simulink model "Flight_Controllers"  (R2024a)
settings: Solver=VariableStepAuto  StartTime=0.0  StopTime=tFinal  FixedStep=0.02  RelTol=1e-3
values from neighbouring files (symbols this model uses):
  bOmega = -bThrust/mThrust    (= 168.963839792)    [Load_VehicleParams.m]
  Cant_cosine_Loss = cos(fanCantAngle)    [Load_VehicleParams.m]
  g = 9.807    [Load_VehicleParams.m]
  g_Offset = 5/6    (= 0.833333333333)    [Load_VehicleParams.m]
  Kd_LatPos = -0.04577    [Load_Controller_Gains_1.m]    (also in Load_Controller_Gains_13.m = -0.1; Load_Controller_Gains_2.m = 0.642; Load_Controller_Gains_3.m = -0.103; Load_Controller_Gains_4.m = 0)
  Kd_LatVel = 0    [Load_Controller_Gains_4.m]
  Kd_Pitch = 14.4    [Load_Controller_Gains_1.m]    (also in Load_Controller_Gains_13.m = 40; Load_Controller_Gains_2.m = 33; Load_Controller_Gains_3.m = 40; Load_Controller_Gains_4.m = 78.1)
  Ki_LatPos = -9.22e-6    (= -9.22e-06)    [Load_Controller_Gains_1.m]    (also in Load_Controller_Gains_13.m = 0.001; Load_Controller_Gains_2.m = 0.0199; Load_Controller_Gains_3.m = 0; Load_Controller_Gains_4.m = 0)
  Ki_LatVel = -0.00284    [Load_Controller_Gains_1.m]    (also in Load_Controller_Gains_2.m = -0.0122; Load_Controller_Gains_4.m = 0)
  Ki_Pitch = 3.17    [Load_Controller_Gains_4.m]
  Kp_LatPos = -0.0024    [Load_Controller_Gains_1.m]    (also in Load_Controller_Gains_13.m = -0.0248; Load_Controller_Gains_2.m = 1.53; Load_Controller_Gains_3.m = -0.0175; Load_Controller_Gains_4.m = 0.413)
  Kp_LatVel = -0.0296    [Load_Controller_Gains_1.m]    (also in Load_Controller_Gains_2.m = -0.059; Load_Controller_Gains_4.m = -0.291)
  Kp_Pitch = 5.36    [Load_Controller_Gains_1.m]    (also in Load_Controller_Gains_13.m = 38; Load_Controller_Gains_2.m = 24.8; Load_Controller_Gains_3.m = 38; Load_Controller_Gains_4.m = 43.7)
  mOmega = 1/mThrust    (= 1.62153397114)    [Load_VehicleParams.m]
  N_LatPos = 54.3    [Load_Controller_Gains_1.m]    (also in Load_Controller_Gains_13.m = 120; Load_Controller_Gains_2.m = 15.8; Load_Controller_Gains_3.m = 12; Load_Controller_Gains_4.m = 0)
  N_LatVel = 0    [Load_Controller_Gains_4.m]
  N_Pitch = 18.2    [Load_Controller_Gains_1.m]    (also in Load_Controller_Gains_13.m = 550; Load_Controller_Gains_2.m = 109; Load_Controller_Gains_3.m = 550; Load_Controller_Gains_4.m = 1115)
  nFans = 4    [Load_VehicleParams.m]
  pitch_Cmd_Limit = 7*pi/180    (= 0.12217304764)    [Load_Controller_Gains_13.m]    (also in Load_Controller_Gains_2.m = 0.10471975512; Load_Controller_Gains_3.m; Load_Controller_Gains_4.m)
  tau_LatPos = 0.2    [Load_Controller_Gains_1.m]    (also in Load_Controller_Gains_2.m = 0.01)
  tau_vCmd = 0.01    [Load_Controller_Gains_2.m]    (also in Load_Controller_Gains_4.m = 0.1)
  tau_xCmd = 0.2    [Load_Controller_Gains_3.m]
  Ts_Control = 1/50    (= 0.02)    [run_Lander_GNC_MonteCarloSim.m]
  vCmd_Integr_Limit = 0.25    [Load_Controller_Gains_2.m]
  velCmd_Limit = 2    [Load_Controller_Gains_2.m]    (also in Load_Controller_Gains_4.m = 0.12217304764)
undefined symbols (not defined in the file or in its folder): den_Gc_z_Pitch, den_Gc_z_Pos, num_Gc_z_Pitch, num_Gc_z_Pos, posCntrl_Integr_Limit
libraries: slpidlib x17
(part 1 of 3)
settings Model: Creator=mhannan  LastModifiedBy=mhann
settings SolverCC: AlgebraicLoopSolver=TrustRegion
settings DataIOCC: SaveOutput=off  SaveTime=off
settings OptimizationCC: DefaultParameterBehavior=Inlined  EnhancedBackFolding=on  PassReuseOutputArgsThreshold=0  OptimizeBlockOrder=speed  DifferentSizesBufferReuse=on
settings DebuggingCC: ParameterTunabilityLossMsg=error  UnconnectedInputMsg=warning  UnconnectedOutputMsg=warning  UnconnectedLineMsg=warning  ArithmeticOperatorsInVariantConditions=warning
settings ModelReferenceCC: EnableRefExpFcnMdlSchedulingChecks=on
settings SFSimCC: SimUseLocalCustomCode=off  MATLABDynamicMemAlloc=off  CustomCodeUndefinedFunction=UseInterfaceOnly
settings RTWCC: RTWUseLocalCustomCode=off  GPUComputeCapability=3.5
settings CodeAppCC: ForceParamTrailComments=on  OperatorAnnotations=on

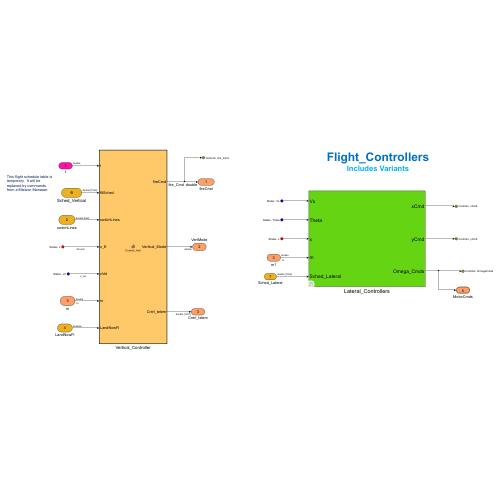
[thumbnail: Simulink's stored preview of the top-level diagram]
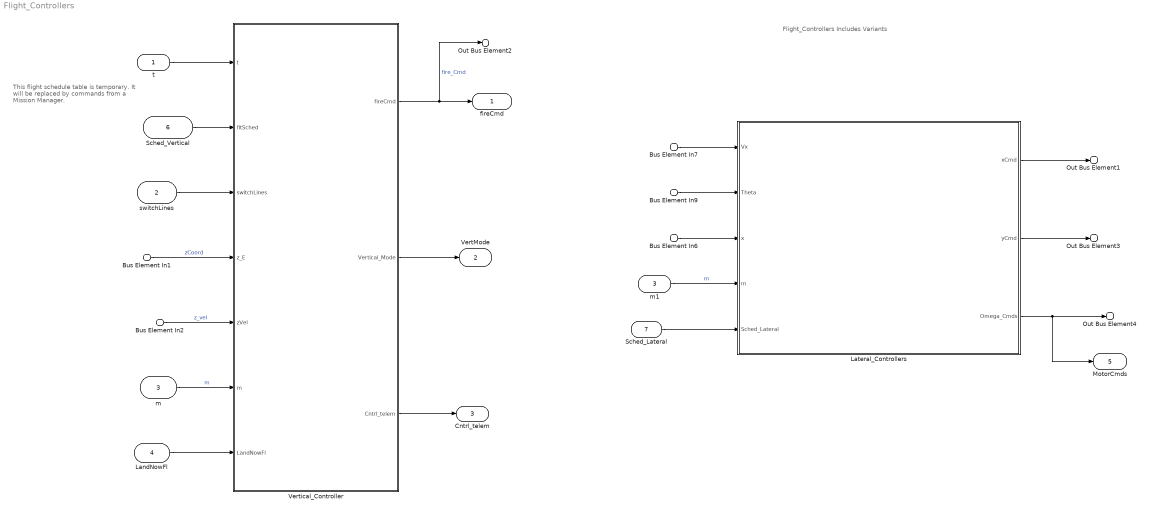
== system Flight_Controllers ==
  note: Flight_Controllers
      | Includes Variants
  note: This flight schedule table is temporary. It will be replaced by commands from a Mission Manager.
  t : Inport  OutDataTypeStr=double  PortDimensions=1  SampleTime=[0.02,0]
  switchLines : Inport  Port=2  OutDataTypeStr=double  PortDimensions=[8 2]
  m : Inport  Port=3  OutDataTypeStr=double  PortDimensions=1
  LandNowFl : Inport  Port=4  OutDataTypeStr=boolean  PortDimensions=1
  Bus Element In6 : Inport  Port=5  PortName=States  Element=x
  Bus Element In7 : Inport  Port=5  PortName=States  Element=VxE
  Bus Element In9 : Inport  Port=5  PortName=States  Element=Theta
  Bus Element In1 : Inport  Port=5  PortName=States  Element=z
  Bus Element In2 : Inport  Port=5  PortName=States  Element=VzB
  Sched_Vertical : Inport  Port=6  OutDataTypeStr=double  PortDimensions=[10 3]
  Sched_Lateral : Inport  Port=7  OutDataTypeStr=double  PortDimensions=[10 4]
  Lateral_Controllers : Subsystem  Variant=on
  Vertical_Controller : MATLAB Function  TreatAsAtomicUnit=on  SystemSampleTime=Ts_Control
  m1 : InportShadow  Port=3  OutDataTypeStr=double  PortDimensions=1
  fireCmd : Outport  OutDataTypeStr=double  PortDimensions=1  SampleTime=[0.02,0]
  VertMode : Outport  Port=2  OutDataTypeStr=double  SampleTime=[0.02,0]
  Cntrl_telem : Outport  Port=3  OutDataTypeStr=double  PortDimensions=[1 10]  SampleTime=[0.02,0]
  Out Bus Element1 : Outport  Port=4  PortName=Controls  Element=xCmd
  Out Bus Element2 : Outport  Port=4  PortName=Controls  Element=fire_Cmd
  Out Bus Element3 : Outport  Port=4  PortName=Controls  Element=yCmd
  Out Bus Element4 : Outport  Port=4  PortName=Controls  Element=OmegaCmds
  MotorCmds : Outport  Port=5  OutDataTypeStr=Bus: MotorCmd_Bus
  wires:
  switchLines/1 -> Vertical_Controller/3(switchLines)
  m/1 -> Vertical_Controller/6(m)  "m"
  LandNowFl/1 -> Vertical_Controller/7(LandNowFl)
  Vertical_Controller/1(fireCmd) -> fireCmd/1, Out Bus Element2/1  "fire_Cmd"
  Vertical_Controller/3(Cntrl_telem) -> Cntrl_telem/1
  Vertical_Controller/2(Vertical_Mode) -> VertMode/1
  t/1 -> Vertical_Controller/1(t)
  Sched_Vertical/1 -> Vertical_Controller/2(fltSched)
  Bus Element In7/1 -> Lateral_Controllers/1(Vx)
  Bus Element In9/1 -> Lateral_Controllers/2(Theta)
  Bus Element In6/1 -> Lateral_Controllers/3(x)
  m1/1 -> Lateral_Controllers/4(m)  "m"
  Sched_Lateral/1 -> Lateral_Controllers/5(Sched_Lateral)
  Bus Element In1/1 -> Vertical_Controller/4(z_E)  "zCoord"
  Bus Element In2/1 -> Vertical_Controller/5(zVel)  "z_vel"
  Lateral_Controllers/1(xCmd) -> Out Bus Element1/1
  Lateral_Controllers/3(Omega_Cmds) -> MotorCmds/1, Out Bus Element4/1
  Lateral_Controllers/2(yCmd) -> Out Bus Element3/1

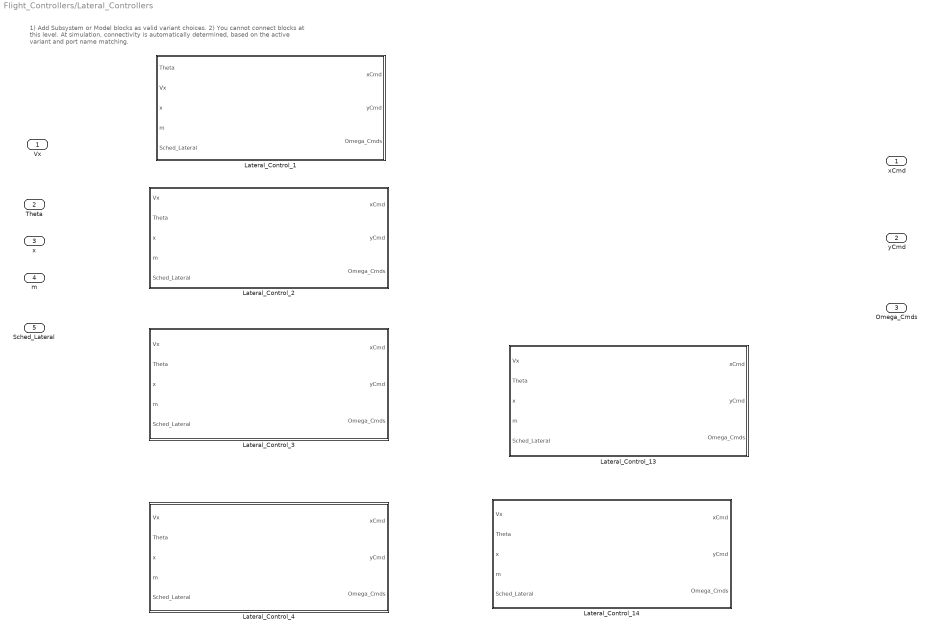
== system Flight_Controllers/Lateral_Controllers ==
  note: 1) Add Subsystem or Model blocks as valid variant choices.
      | 2) You cannot connect blocks at this level. At simulation, connectivity is automatically
      | determined, based on the active variant and port name matching.
  Vx : Inport
  Theta : Inport  Port=2
  x : Inport  Port=3
  m : Inport  Port=4
  Sched_Lateral : Inport  Port=5
  Lateral_Control_1 : Subsystem  VariantControl=LatCntrl_variant == 1
  Lateral_Control_13 : Subsystem  VariantControl=LatCntrl_variant == 13
  Lateral_Control_14 : Subsystem  VariantControl=LatCntrl_variant == 14
  Lateral_Control_2 : Subsystem  VariantControl=LatCntrl_variant == 2
  Lateral_Control_3 : Subsystem  VariantControl=LatCntrl_variant == 3
  Lateral_Control_4 : Subsystem  VariantControl=LatCntrl_variant == 4
  xCmd : Outport
  yCmd : Outport  Port=2
  Omega_Cmds : Outport  Port=3

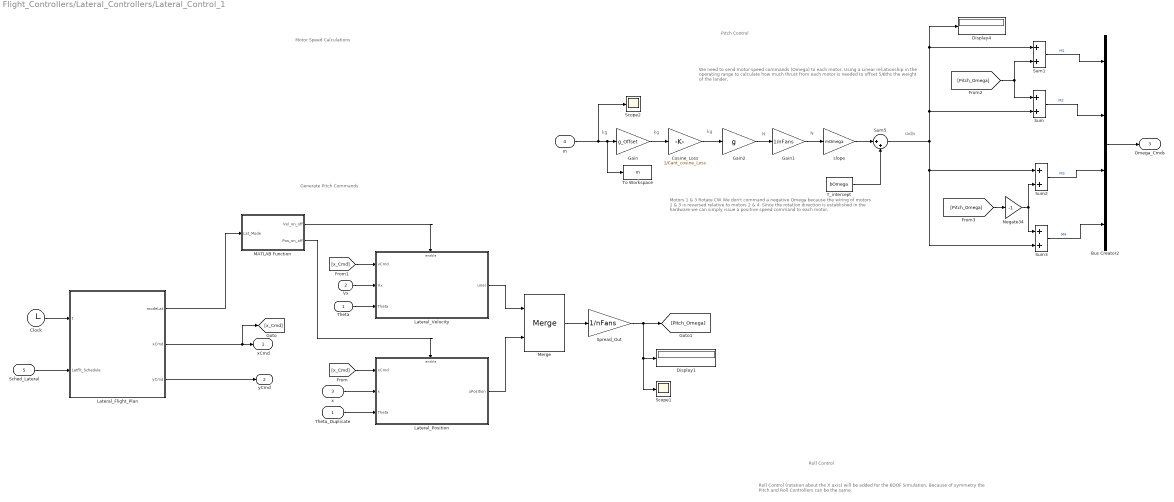
== system Flight_Controllers/Lateral_Controllers/Lateral_Control_1 ==
  note: Roll Control (rotation about the X axis) will be added for the 6DOF Simulation. Because of symmetry the Pitch and Roll Controllers can be the same.
  note: N
  note: Motors 1 & 3 Rotate CW
      | We don't command a negative Omega because the
      | wiring of motors 1 & 3 is reversed relative to motors 2 & 4.
      |
      | Since the rotation direction is established in the hardware
      | we can simply issue a positive speed command to each motor.
  note: We need to send motor speed commands (Omega) to each motor.
      |
      | Using a Linear rel;ationship in the operating range to calculate how much thrust from each motor is needed to offset 5/6ths the weight of the lander.
  note: Motor Speed Calculations
  note: kg
  note: kg
  note: N
  note: kg
  note: rad/s
  note: Pitch Control
  note: Roll Control
  note: Generate Pitch Commands
  Theta : Inport
  Vx : Inport  Port=2
  x : Inport  Port=3
  m : Inport  Port=4
  Sched_Lateral : Inport  Port=5
  Bus Creator2 : BusCreator  Inputs=4  OutDataTypeStr=Bus: MotorCmd_Bus
  Clock : Clock
  Cosine_Loss : Gain  Gain=1/Cant_cosine_Loss
  Display1 : Display
  Display4 : Display
  Gain : Gain  Gain=g_Offset
  Gain1 : Gain  Gain=1/nFans
  Gain2 : Gain  Gain=g
  Lateral_Flight_Plan : MATLAB Function  TreatAsAtomicUnit=on
  Lateral_Position : Subsystem  TreatAsAtomicUnit=on
  Lateral_Velocity : Subsystem  TreatAsAtomicUnit=on
  MATLAB Function : MATLAB Function  TreatAsAtomicUnit=on
  Merge : Merge
  Negate34 : Gain  Gain=-1
  Scope1 : Scope
  Scope2 : Scope
  Spread_Out : Gain  Gain=1/nFans
  Sum{,1..3} (4 alike) : Sum
  Sum5 : Sum  Inputs=|++
  Theta_Duplicate : InportShadow
  To Workspace : ToWorkspace  VariableName=m  SaveFormat=Timeseries  SampleTime=-1
  Y_intercept : Constant  Value=bOmega
  slope : Gain  Gain=mOmega
  xCmd : Outport
  yCmd : Outport  Port=2
  Omega_Cmds : Outport  Port=3
  wires:
  MATLAB Function/1(Vel_on_off) -> Lateral_Velocity/Enable
  MATLAB Function/2(Pos_on_off) -> Lateral_Position/Enable
  [x_Cmd] -> Lateral_Velocity/1(vCmd)
  Lateral_Position/1(uPosition) -> Merge/2
  Clock/1 -> Lateral_Flight_Plan/1(t)
  Lateral_Flight_Plan/2(xCmd) -> xCmd/1, [x_Cmd]
  Lateral_Flight_Plan/1(modeLat) -> MATLAB Function/1(Lat_Mode)
  [x_Cmd] -> Lateral_Position/1(xCmd)
  Merge/1 -> Spread_Out/1
  Lateral_Velocity/1(uVel) -> Merge/1
  Vx/1 -> Lateral_Velocity/2(Vx)
  Lateral_Flight_Plan/3(yCmd) -> yCmd/1
  x/1 -> Lateral_Position/2(x)
  Theta/1 -> Lateral_Velocity/3(Theta)
  Theta_Duplicate/1 -> Lateral_Position/3(Theta)
  Gain2/1 -> Gain1/1
  Sum3/1 -> Bus Creator2/4  "M4"
  Negate34/1 -> Sum3/1, Sum2/2
  Gain1/1 -> slope/1
  Bus Creator2/1 -> Omega_Cmds/1
  slope/1 -> Sum5/1
  Sum1/1 -> Bus Creator2/1  "M1"
  Sum5/1 -> Sum3/2, Sum2/1, Display4/1, Sum1/1, Sum/2
  Y_intercept/1 -> Sum5/2
  Sum/1 -> Bus Creator2/2  "M2"
  m/1 -> Scope2/1, To Workspace/1, Gain/1
  Cosine_Loss/1 -> Gain2/1
  Gain/1 -> Cosine_Loss/1
  Spread_Out/1 -> Display1/1, Scope1/1, [Pitch_Omega]
  [Pitch_Omega] -> Sum/1, Sum1/2
  Sum2/1 -> Bus Creator2/3  "M3"
  [Pitch_Omega] -> Negate34/1
  Sched_Lateral/1 -> Lateral_Flight_Plan/2(LatFlt_Schedule)

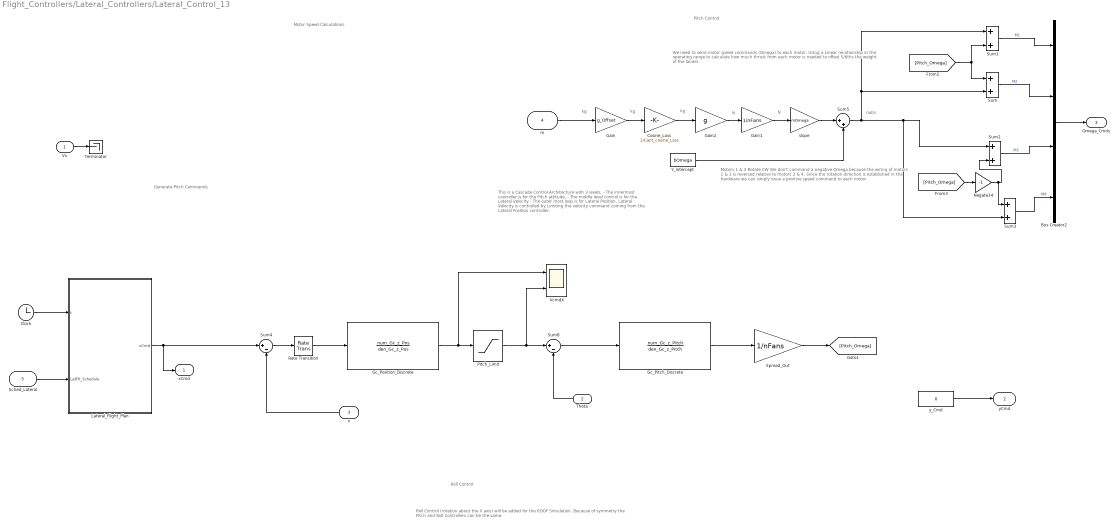
== system Flight_Controllers/Lateral_Controllers/Lateral_Control_13 ==
  note: Roll Control (rotation about the X axis) will be added for the 6DOF Simulation. Because of symmetry the Pitch and Roll Controllers can be the same.
  note: N
  note: Motors 1 & 3 Rotate CW
      | We don't command a negative Omega because the
      | wiring of motors 1 & 3 is reversed relative to motors 2 & 4.
      |
      | Since the rotation direction is established in the hardware
      | we can simply issue a positive speed command to each motor.
  note: We need to send motor speed commands (Omega) to each motor.
      |
      | Using a Linear rel;ationship in the operating range to calculate how much thrust from each motor is needed to offset 5/6ths the weight of the lander.
  note: Motor Speed Calculations
  note: kg
  note: kg
  note: N
  note: kg
  note: rad/s
  note: Pitch Control
  note: Roll Control
  note: Generate Pitch Commands
  note: This is a Cascade Control Architecture with 3 levels.
      | - The innermost controller is for the Pitch attitude.
      | - The middle level control is for the Lateral Velocity
      | - The outer most loop is for Lateral Position.
      | Lateral Velocity is controlled by Limiting the velocity command coming from the Lateral Position controller.
  Vx : Inport
  Theta : Inport  Port=2
  x : Inport  Port=3
  m : Inport  Port=4
  Sched_Lateral : Inport  Port=5
  Bus Creator2 : BusCreator  Inputs=4  OutDataTypeStr=Bus: MotorCmd_Bus
  Clock : Clock
  Cosine_Loss : Gain  Gain=1/Cant_cosine_Loss
  Gain : Gain  Gain=g_Offset
  Gain1 : Gain  Gain=1/nFans
  Gain2 : Gain  Gain=g
  Gc_Pitch_Discrete : DiscreteTransferFcn  Numerator=num_Gc_z_Pitch  Denominator=den_Gc_z_Pitch
  Gc_Position_Discrete : DiscreteTransferFcn  Numerator=num_Gc_z_Pos  Denominator=den_Gc_z_Pos
  Lateral_Flight_Plan : MATLAB Function  TreatAsAtomicUnit=on
  Negate34 : Gain  Gain=-1
  Pitch_Limit : Saturate  UpperLimit=pitch_Cmd_Limit  LowerLimit=-pitch_Cmd_Limit
  Rate Transition : RateTransition  OutPortSampleTime=T
  Spread_Out : Gain  Gain=1/nFans
  Sum{,1..3} (4 alike) : Sum
  Sum4 : Sum  Inputs=|+-
  Sum5 : Sum  Inputs=|++
  Sum8 : Sum  Inputs=|+-
  Terminator : Terminator
  VcmdX : Scope  NumInputPorts=2
  Y_intercept : Constant  Value=bOmega
  slope : Gain  Gain=mOmega
  y_Cmd : Constant  Value=0
  xCmd : Outport
  yCmd : Outport  Port=2
  Omega_Cmds : Outport  Port=3
  wires:
  Clock/1 -> Lateral_Flight_Plan/1(t)
  Gain2/1 -> Gain1/1
  Sum3/1 -> Bus Creator2/4  "M4"
  Negate34/1 -> Sum3/1, Sum2/2
  Gain1/1 -> slope/1
  Bus Creator2/1 -> Omega_Cmds/1
  slope/1 -> Sum5/1
  Sum1/1 -> Bus Creator2/1  "M1"
  Sum5/1 -> Sum3/2, Sum2/1, Sum1/1, Sum/2
  Y_intercept/1 -> Sum5/2
  Sum/1 -> Bus Creator2/2  "M2"
  m/1 -> Gain/1
  Cosine_Loss/1 -> Gain2/1
  Gain/1 -> Cosine_Loss/1
  Spread_Out/1 -> [Pitch_Omega]
  [Pitch_Omega] -> Sum/1, Sum1/2
  Sum2/1 -> Bus Creator2/3  "M3"
  [Pitch_Omega] -> Negate34/1
  Sched_Lateral/1 -> Lateral_Flight_Plan/2(LatFlt_Schedule)
  Lateral_Flight_Plan/1(xCmd) -> Sum4/1, xCmd/1
  x/1 -> Sum4/2
  Vx/1 -> Terminator/1
  Theta/1 -> Sum8/2
  Gc_Position_Discrete/1 -> VcmdX/1, Pitch_Limit/1
  Pitch_Limit/1 -> VcmdX/2, Sum8/1
  Sum8/1 -> Gc_Pitch_Discrete/1
  y_Cmd/1 -> yCmd/1
  Gc_Pitch_Discrete/1 -> Spread_Out/1
  Sum4/1 -> Rate Transition/1
  Rate Transition/1 -> Gc_Position_Discrete/1

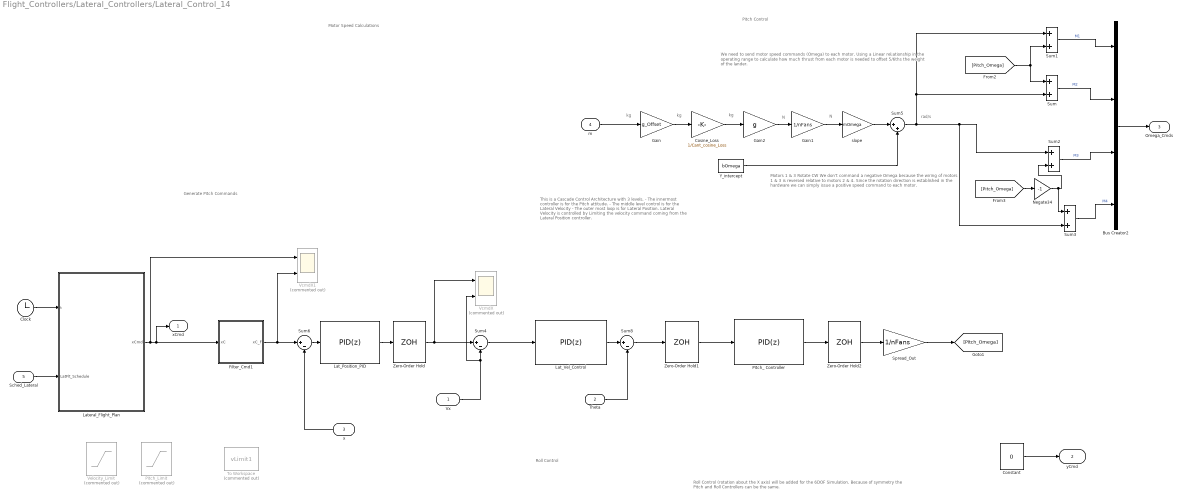
== system Flight_Controllers/Lateral_Controllers/Lateral_Control_14 ==
  note: kg
  note: kg
  note: N
  note: Motor Speed Calculations
  note: We need to send motor speed commands (Omega) to each motor.
      |
      | Using a Linear rel;ationship in the operating range to calculate how much thrust from each motor is needed to offset 5/6ths the weight of the lander.
  note: Motors 1 & 3 Rotate CW
      | We don't command a negative Omega because the
      | wiring of motors 1 & 3 is reversed relative to motors 2 & 4.
      |
      | Since the rotation direction is established in the hardware
      | we can simply issue a positive speed command to each motor.
  note: Roll Control (rotation about the X axis) will be added for the 6DOF Simulation. Because of symmetry the Pitch and Roll Controllers can be the same.
  note: N
  note: kg
  note: Roll Control
  note: rad/s
  note: Generate Pitch Commands
  note: This is a Cascade Control Architecture with 3 levels.
      | - The innermost controller is for the Pitch attitude.
      | - The middle level control is for the Lateral Velocity
      | - The outer most loop is for Lateral Position.
      | Lateral Velocity is controlled by Limiting the velocity command coming from the Lateral Position controller.
  note: Pitch Control
  Vx : Inport
  Theta : Inport  Port=2
  x : Inport  Port=3
  m : Inport  Port=4
  Sched_Lateral : Inport  Port=5
  Bus Creator2 : BusCreator  Inputs=4  OutDataTypeStr=Bus: MotorCmd_Bus
  Clock : Clock
  Constant : Constant  Value=0
  Cosine_Loss : Gain  Gain=1/Cant_cosine_Loss
  Filter_Cmd1 : Subsystem
  Gain : Gain  Gain=g_Offset
  Gain1 : Gain  Gain=1/nFans
  Gain2 : Gain  Gain=g
  Lat_Position_PID : slpidlib/PID Controller  Controller=PID  Form=Parallel  TimeDomain=Discrete-time  UseExternalTs=off  SampleTime=0.02  IntegratorMethod=Forward Euler  FilterMethod=Forward Euler  ControllerParametersSource=internal  P=Kp_LatPos  I=Ki_LatPos  UseKiTs=off  D=Kd_LatPos  UseExternalDerivativeSource=off  N=N_LatPos  UseFilter=on  TunerSelectOption=Transfer Function Based (PID Tuner App)  InitialConditionSource=internal  InitialConditionForIntegrator=0  InitialConditionForFilter=0  DifferentiatorICPrevScaledInput=0  ExternalReset=none  TrackingMode=off  Kt=1  LimitOutput=off  SatLimitsSource=internal  UpperSaturationLimit=inf  LowerSaturationLimit=-inf  LinearizeAsGain=on  AntiWindupMode=none  Kb=1  LimitIntegrator=off  UpperIntegratorSaturationLimit=vCmd_Integr_Limit  LowerIntegratorSaturationLimit=-vCmd_Integr_Limit  POutMin=[]  POutMax=[]  IOutMin=[]  IOutMax=[]  DOutMin=[]  DOutMax=[]  NOutMin=[]  NOutMax=[]  SumOutMin=[]  SumOutMax=[]  SaturationOutMin=[]  SaturationOutMax=[]  PParamMin=[]  PParamMax=[]  IParamMin=[]  IParamMax=[]  DParamMin=[]  DParamMax=[]  NParamMin=[]  NParamMax=[]  KbParamMin=[]  KbParamMax=[]  KtParamMin=[]  KtParamMax=[]  KbOutMin=[]  KbOutMax=[]  KtOutMin=[]  KtOutMax=[]  IntegratorOutMin=[]  IntegratorOutMax=[]  FilterOutMin=[]  FilterOutMax=[]  SumI1OutMin=[]  SumI1OutMax=[]  SumI2OutMin=[]  SumI2OutMax=[]  SumI3OutMin=[]  SumI3OutMax=[]  SumI4OutMin=[]  SumI4OutMax=[]  SumDOutMin=[]  SumDOutMax=[]  DifferentiatorOutMin=[]  DifferentiatorOutMax=[]  FilterDiffOutCoefMin=[]  FilterDiffOutCoefMax=[]  ReciprocalOutMin=[]  ReciprocalOutMax=[]  SumDenOutMin=[]  SumDenOutMax=[]  SumNumOutMin=[]  SumNumOutMax=[]  DivideOutMin=[]  DivideOutMax=[]  UdiffTsProdOutMin=[]  UdiffTsProdOutMax=[]  NTsProdOutMin=[]  NTsProdOutMax=[]  UintegralTsProdOutMin=[]  UintegralTsProdOutMax=[]  UngainTsProdOutMin=[]  UngainTsProdOutMax=[]  ClampingZeroOutDataTypeStr=Inherit: Inherit via back propagation  ClampingZeroOutMin=[]  ClampingZeroOutMax=[]  FilterDenConstantOutDataTypeStr=Inherit: Inherit via back propagation  FilterDenConstantOutMin=[]  FilterDenConstantOutMax=[]  PCopyOutDataTypeStr=Inherit: Inherit via back propagation  PCopyOutMin=[]  PCopyOutMax=[]  NCopyOutDataTypeStr=Inherit: Inherit via back propagation  NCopyOutMin=[]  NCopyOutMax=[]  IntegratorContinuousStateAttributes=''  IntegratorStateMustResolveToSignalObject=off  IntegratorRTWStateStorageClass=Auto  FilterContinuousStateAttributes=''  FilterStateMustResolveToSignalObject=off  FilterRTWStateStorageClass=Auto  ParallelPVariant=InternalParameters  IdealPVariant=Disabled  IVariant=InternalParameters  DVariant=InternalParameters  IntegratorVariant=Discrete  SatVariant=Disabled  AWVariant=Passthrough  PCopyVariant=Disabled  TRVariant=Disabled  FdbkBlocksVariant=Forward  IdealPFdbkVariant=Disabled  SatFdbkVariant=Disabled  DerivativeFilterVariant=ForwardEulerFilter  NVariant=InternalParameters  NCopyVariant=Disabled  FilterICVariant=InternalICsFilter  IntegratorICVariant=InternalICs  ExternalResetVariant=Disabled  TRSumVariant=Passthrough  SumFdbkVariant=Disabled  SumVariant=Sum_PID  TsampFilterVariant=InternalTs  TsampNgainVariant=Passthrough  TsampIntegralVariant=Disabled_SignalSpec  ExternalSaturationOutDataTypeStr=Inherit: Same as second input  DerivativeSourceVariant=ErrorSignal
  Lat_Vel_Control : slpidlib/PID Controller  Controller=PID  Form=Parallel  TimeDomain=Discrete-time  UseExternalTs=off  SampleTime=0.02  IntegratorMethod=Forward Euler  FilterMethod=Forward Euler  ControllerParametersSource=internal  P=Kp_LatVel  I=Ki_LatVel  UseKiTs=off  D=Kd_LatVel  UseExternalDerivativeSource=off  N=N_LatVel  UseFilter=on  TunerSelectOption=Transfer Function Based (PID Tuner App)  InitialConditionSource=internal  InitialConditionForIntegrator=0  InitialConditionForFilter=0  DifferentiatorICPrevScaledInput=0  ExternalReset=none  TrackingMode=off  Kt=1  LimitOutput=off  SatLimitsSource=internal  UpperSaturationLimit=inf  LowerSaturationLimit=-inf  LinearizeAsGain=on  AntiWindupMode=none  Kb=1  LimitIntegrator=off  UpperIntegratorSaturationLimit=inf  LowerIntegratorSaturationLimit=-inf  POutMin=[]  POutMax=[]  IOutMin=[]  IOutMax=[]  DOutMin=[]  DOutMax=[]  NOutMin=[]  NOutMax=[]  SumOutMin=[]  SumOutMax=[]  SaturationOutMin=[]  SaturationOutMax=[]  PParamMin=[]  PParamMax=[]  IParamMin=[]  IParamMax=[]  DParamMin=[]  DParamMax=[]  NParamMin=[]  NParamMax=[]  KbParamMin=[]  KbParamMax=[]  KtParamMin=[]  KtParamMax=[]  KbOutMin=[]  KbOutMax=[]  KtOutMin=[]  KtOutMax=[]  IntegratorOutMin=[]  IntegratorOutMax=[]  FilterOutMin=[]  FilterOutMax=[]  SumI1OutMin=[]  SumI1OutMax=[]  SumI2OutMin=[]  SumI2OutMax=[]  SumI3OutMin=[]  SumI3OutMax=[]  SumI4OutMin=[]  SumI4OutMax=[]  SumDOutMin=[]  SumDOutMax=[]  DifferentiatorOutMin=[]  DifferentiatorOutMax=[]  FilterDiffOutCoefMin=[]  FilterDiffOutCoefMax=[]  ReciprocalOutMin=[]  ReciprocalOutMax=[]  SumDenOutMin=[]  SumDenOutMax=[]  SumNumOutMin=[]  SumNumOutMax=[]  DivideOutMin=[]  DivideOutMax=[]  UdiffTsProdOutMin=[]  UdiffTsProdOutMax=[]  NTsProdOutMin=[]  NTsProdOutMax=[]  UintegralTsProdOutMin=[]  UintegralTsProdOutMax=[]  UngainTsProdOutMin=[]  UngainTsProdOutMax=[]  ClampingZeroOutDataTypeStr=Inherit: Inherit via back propagation  ClampingZeroOutMin=[]  ClampingZeroOutMax=[]  FilterDenConstantOutDataTypeStr=Inherit: Inherit via back propagation  FilterDenConstantOutMin=[]  FilterDenConstantOutMax=[]  PCopyOutDataTypeStr=Inherit: Inherit via back propagation  PCopyOutMin=[]  PCopyOutMax=[]  NCopyOutDataTypeStr=Inherit: Inherit via back propagation  NCopyOutMin=[]  NCopyOutMax=[]  IntegratorContinuousStateAttributes=''  IntegratorStateMustResolveToSignalObject=off  IntegratorRTWStateStorageClass=Auto  FilterContinuousStateAttributes=''  FilterStateMustResolveToSignalObject=off  FilterRTWStateStorageClass=Auto  ParallelPVariant=InternalParameters  IdealPVariant=Disabled  IVariant=InternalParameters  DVariant=InternalParameters  IntegratorVariant=Discrete  SatVariant=Disabled  AWVariant=Passthrough  PCopyVariant=Disabled  TRVariant=Disabled  FdbkBlocksVariant=Forward  IdealPFdbkVariant=Disabled  SatFdbkVariant=Disabled  DerivativeFilterVariant=ForwardEulerFilter  NVariant=InternalParameters  NCopyVariant=Disabled  FilterICVariant=InternalICsFilter  IntegratorICVariant=InternalICs  ExternalResetVariant=Disabled  TRSumVariant=Passthrough  SumFdbkVariant=Disabled  SumVariant=Sum_PID  TsampFilterVariant=InternalTs  TsampNgainVariant=Passthrough  TsampIntegralVariant=Disabled_SignalSpec  ExternalSaturationOutDataTypeStr=Inherit: Same as second input  DerivativeSourceVariant=ErrorSignal
  Lateral_Flight_Plan : MATLAB Function  TreatAsAtomicUnit=on
  Negate34 : Gain  Gain=-1
  Pitch_ Controller : slpidlib/PID Controller  Controller=PID  Form=Parallel  TimeDomain=Discrete-time  UseExternalTs=off  SampleTime=0.02  IntegratorMethod=Forward Euler  FilterMethod=Forward Euler  ControllerParametersSource=internal  P=Kp_Pitch  I=Ki_Pitch  UseKiTs=off  D=Kd_Pitch  UseExternalDerivativeSource=off  N=N_Pitch  UseFilter=on  TunerSelectOption=Transfer Function Based (PID Tuner App)  InitialConditionSource=internal  InitialConditionForIntegrator=0  InitialConditionForFilter=0  DifferentiatorICPrevScaledInput=0  ExternalReset=none  TrackingMode=off  Kt=1  LimitOutput=off  SatLimitsSource=internal  UpperSaturationLimit=inf  LowerSaturationLimit=-inf  LinearizeAsGain=on  AntiWindupMode=none  Kb=1  LimitIntegrator=off  UpperIntegratorSaturationLimit=inf  LowerIntegratorSaturationLimit=-inf  POutMin=[]  POutMax=[]  IOutMin=[]  IOutMax=[]  DOutMin=[]  DOutMax=[]  NOutMin=[]  NOutMax=[]  SumOutMin=[]  SumOutMax=[]  SaturationOutMin=[]  SaturationOutMax=[]  PParamMin=[]  PParamMax=[]  IParamMin=[]  IParamMax=[]  DParamMin=[]  DParamMax=[]  NParamMin=[]  NParamMax=[]  KbParamMin=[]  KbParamMax=[]  KtParamMin=[]  KtParamMax=[]  KbOutMin=[]  KbOutMax=[]  KtOutMin=[]  KtOutMax=[]  IntegratorOutMin=[]  IntegratorOutMax=[]  FilterOutMin=[]  FilterOutMax=[]  SumI1OutMin=[]  SumI1OutMax=[]  SumI2OutMin=[]  SumI2OutMax=[]  SumI3OutMin=[]  SumI3OutMax=[]  SumI4OutMin=[]  SumI4OutMax=[]  SumDOutMin=[]  SumDOutMax=[]  DifferentiatorOutMin=[]  DifferentiatorOutMax=[]  FilterDiffOutCoefMin=[]  FilterDiffOutCoefMax=[]  ReciprocalOutMin=[]  ReciprocalOutMax=[]  SumDenOutMin=[]  SumDenOutMax=[]  SumNumOutMin=[]  SumNumOutMax=[]  DivideOutMin=[]  DivideOutMax=[]  UdiffTsProdOutMin=[]  UdiffTsProdOutMax=[]  NTsProdOutMin=[]  NTsProdOutMax=[]  UintegralTsProdOutMin=[]  UintegralTsProdOutMax=[]  UngainTsProdOutMin=[]  UngainTsProdOutMax=[]  ClampingZeroOutDataTypeStr=Inherit: Inherit via back propagation  ClampingZeroOutMin=[]  ClampingZeroOutMax=[]  FilterDenConstantOutDataTypeStr=Inherit: Inherit via back propagation  FilterDenConstantOutMin=[]  FilterDenConstantOutMax=[]  PCopyOutDataTypeStr=Inherit: Inherit via back propagation  PCopyOutMin=[]  PCopyOutMax=[]  NCopyOutDataTypeStr=Inherit: Inherit via back propagation  NCopyOutMin=[]  NCopyOutMax=[]  IntegratorContinuousStateAttributes=''  IntegratorStateMustResolveToSignalObject=off  IntegratorRTWStateStorageClass=Auto  FilterContinuousStateAttributes=''  FilterStateMustResolveToSignalObject=off  FilterRTWStateStorageClass=Auto  ParallelPVariant=InternalParameters  IdealPVariant=Disabled  IVariant=InternalParameters  DVariant=InternalParameters  IntegratorVariant=Discrete  SatVariant=Disabled  AWVariant=Passthrough  PCopyVariant=Disabled  TRVariant=Disabled  FdbkBlocksVariant=Forward  IdealPFdbkVariant=Disabled  SatFdbkVariant=Disabled  DerivativeFilterVariant=ForwardEulerFilter  NVariant=InternalParameters  NCopyVariant=Disabled  FilterICVariant=InternalICsFilter  IntegratorICVariant=InternalICs  ExternalResetVariant=Disabled  TRSumVariant=Passthrough  SumFdbkVariant=Disabled  SumVariant=Sum_PID  TsampFilterVariant=InternalTs  TsampNgainVariant=Passthrough  TsampIntegralVariant=Disabled_SignalSpec  ExternalSaturationOutDataTypeStr=Inherit: Same as second input  DerivativeSourceVariant=ErrorSignal
  Pitch_Limit : Saturate  Commented=on  UpperLimit=pitch_Cmd_Limit  LowerLimit=-pitch_Cmd_Limit
  Spread_Out : Gain  Gain=1/nFans
  Sum{,1..3} (4 alike) : Sum
  Sum4 : Sum  Inputs=|+-
  Sum5 : Sum  Inputs=|++
  Sum6 : Sum  Inputs=|+-
  Sum8 : Sum  Inputs=|+-
  To Workspace : ToWorkspace  Commented=on  VariableName=vLimit1  SaveFormat=Timeseries  SampleTime=-1
  VcmdX : Scope  Commented=on  NumInputPorts=2
  VcmdX1 : Scope  Commented=on  NumInputPorts=2
  Velocity_Limit : Saturate  Commented=on  UpperLimit=velCmd_Limit  LowerLimit=-velCmd_Limit
  Y_intercept : Constant  Value=bOmega
  Zero-Order Hold : ZeroOrderHold  SampleTime=-1
  Zero-Order Hold1 : ZeroOrderHold  SampleTime=-1
  Zero-Order Hold2 : ZeroOrderHold  SampleTime=-1
  slope : Gain  Gain=mOmega
  xCmd : Outport
  yCmd : Outport  Port=2
  Omega_Cmds : Outport  Port=3
  wires:
  Sum8/1 -> Zero-Order Hold1/1
  Sum/1 -> Bus Creator2/2  "M2"
  m/1 -> Gain/1
  Sched_Lateral/1 -> Lateral_Flight_Plan/2(LatFlt_Schedule)
  Constant/1 -> yCmd/1
  Filter_Cmd1/1(xC_F) -> VcmdX1/2, Sum6/1
  Bus Creator2/1 -> Omega_Cmds/1
  Clock/1 -> Lateral_Flight_Plan/1(t)
  Pitch_ Controller/1 -> Zero-Order Hold2/1
  x/1 -> Sum6/2
  Spread_Out/1 -> [Pitch_Omega]
  Lat_Position_PID/1 -> Zero-Order Hold/1
  [Pitch_Omega] -> Sum/1, Sum1/2
  Sum1/1 -> Bus Creator2/1  "M1"
  Vx/1 -> VcmdX/2, Sum4/2
  Y_intercept/1 -> Sum5/2
  Negate34/1 -> Sum3/1, Sum2/2
  Sum5/1 -> Sum3/2, Sum2/1, Sum1/1, Sum/2
  Theta/1 -> Sum8/2
  slope/1 -> Sum5/1
  Lat_Vel_Control/1 -> Sum8/1
  Sum4/1 -> Lat_Vel_Control/1
  [Pitch_Omega] -> Negate34/1
  ? -> To Workspace/1
  Gain/1 -> Cosine_Loss/1
  Cosine_Loss/1 -> Gain2/1
  Sum2/1 -> Bus Creator2/3  "M3"
  Gain1/1 -> slope/1
  Gain2/1 -> Gain1/1
  Lateral_Flight_Plan/1(xCmd) -> Filter_Cmd1/1(xC), xCmd/1, VcmdX1/1
  Sum3/1 -> Bus Creator2/4  "M4"
  Sum6/1 -> Lat_Position_PID/1
  Zero-Order Hold/1 -> VcmdX/1, Sum4/1
  Zero-Order Hold1/1 -> Pitch_ Controller/1
  Zero-Order Hold2/1 -> Spread_Out/1

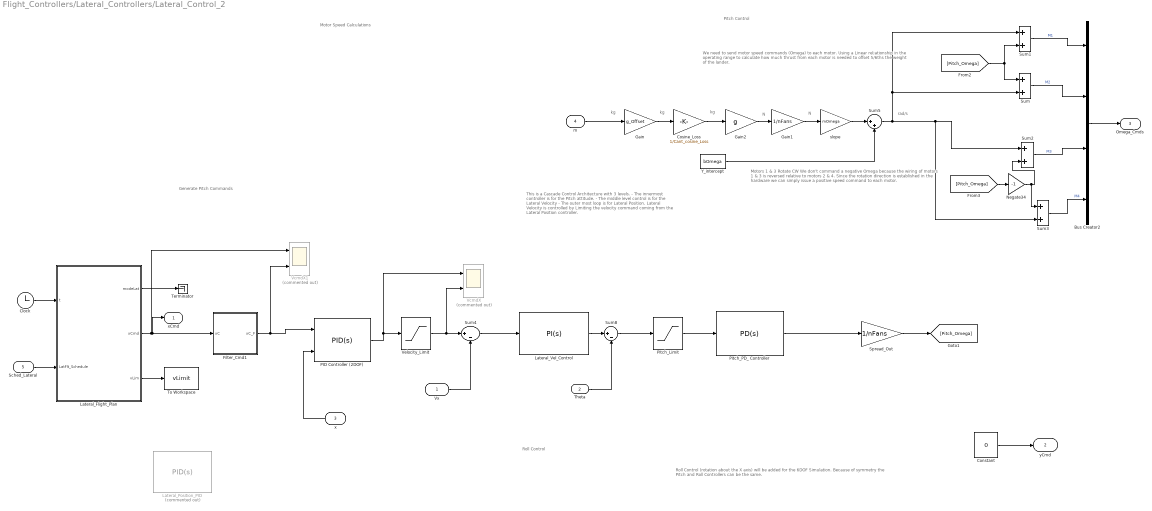
== system Flight_Controllers/Lateral_Controllers/Lateral_Control_2 ==
  note: Roll Control (rotation about the X axis) will be added for the 6DOF Simulation. Because of symmetry the Pitch and Roll Controllers can be the same.
  note: N
  note: Motors 1 & 3 Rotate CW
      | We don't command a negative Omega because the
      | wiring of motors 1 & 3 is reversed relative to motors 2 & 4.
      |
      | Since the rotation direction is established in the hardware
      | we can simply issue a positive speed command to each motor.
  note: We need to send motor speed commands (Omega) to each motor.
      |
      | Using a Linear rel;ationship in the operating range to calculate how much thrust from each motor is needed to offset 5/6ths the weight of the lander.
  note: Motor Speed Calculations
  note: kg
  note: kg
  note: N
  note: kg
  note: rad/s
  note: Pitch Control
  note: Roll Control
  note: Generate Pitch Commands
  note: This is a Cascade Control Architecture with 3 levels.
      | - The innermost controller is for the Pitch attitude.
      | - The middle level control is for the Lateral Velocity
      | - The outer most loop is for Lateral Position.
      | Lateral Velocity is controlled by Limiting the velocity command coming from the Lateral Position controller.
  Vx : Inport
  Theta : Inport  Port=2
  x : Inport  Port=3
  m : Inport  Port=4
  Sched_Lateral : Inport  Port=5
  Bus Creator2 : BusCreator  Inputs=4  OutDataTypeStr=Bus: MotorCmd_Bus
  Clock : Clock
  Constant : Constant  Value=0
  Cosine_Loss : Gain  Gain=1/Cant_cosine_Loss
  Filter_Cmd1 : Subsystem
  Gain : Gain  Gain=g_Offset
  Gain1 : Gain  Gain=1/nFans
  Gain2 : Gain  Gain=g
  Lateral_Flight_Plan : MATLAB Function  TreatAsAtomicUnit=on
  Lateral_Position_PID : slpidlib/PID Controller  Commented=on  Controller=PID  Form=Parallel  TimeDomain=Continuous-time  UseExternalTs=off  SampleTime=-1  IntegratorMethod=Forward Euler  FilterMethod=Forward Euler  ControllerParametersSource=internal  P=Kp_LatPos  I=Ki_LatPos  UseKiTs=off  D=Kd_LatPos  UseExternalDerivativeSource=off  N=N_LatPos  UseFilter=on  TunerSelectOption=Transfer Function Based (PID Tuner App)  InitialConditionSource=internal  InitialConditionForIntegrator=0  InitialConditionForFilter=0  DifferentiatorICPrevScaledInput=0  ExternalReset=none  TrackingMode=off  Kt=1  LimitOutput=off  SatLimitsSource=internal  UpperSaturationLimit=inf  LowerSaturationLimit=-inf  LinearizeAsGain=on  AntiWindupMode=none  Kb=1  LimitIntegrator=on  UpperIntegratorSaturationLimit=vCmd_Integr_Limit  LowerIntegratorSaturationLimit=-vCmd_Integr_Limit  POutMin=[]  POutMax=[]  IOutMin=[]  IOutMax=[]  DOutMin=[]  DOutMax=[]  NOutMin=[]  NOutMax=[]  SumOutMin=[]  SumOutMax=[]  SaturationOutMin=[]  SaturationOutMax=[]  PParamMin=[]  PParamMax=[]  IParamMin=[]  IParamMax=[]  DParamMin=[]  DParamMax=[]  NParamMin=[]  NParamMax=[]  KbParamMin=[]  KbParamMax=[]  KtParamMin=[]  KtParamMax=[]  KbOutMin=[]  KbOutMax=[]  KtOutMin=[]  KtOutMax=[]  IntegratorOutMin=[]  IntegratorOutMax=[]  FilterOutMin=[]  FilterOutMax=[]  SumI1OutMin=[]  SumI1OutMax=[]  SumI2OutMin=[]  SumI2OutMax=[]  SumI3OutMin=[]  SumI3OutMax=[]  SumI4OutMin=[]  SumI4OutMax=[]  SumDOutMin=[]  SumDOutMax=[]  DifferentiatorOutMin=[]  DifferentiatorOutMax=[]  FilterDiffOutCoefMin=[]  FilterDiffOutCoefMax=[]  ReciprocalOutMin=[]  ReciprocalOutMax=[]  SumDenOutMin=[]  SumDenOutMax=[]  SumNumOutMin=[]  SumNumOutMax=[]  DivideOutMin=[]  DivideOutMax=[]  UdiffTsProdOutMin=[]  UdiffTsProdOutMax=[]  NTsProdOutMin=[]  NTsProdOutMax=[]  UintegralTsProdOutMin=[]  UintegralTsProdOutMax=[]  UngainTsProdOutMin=[]  UngainTsProdOutMax=[]  ClampingZeroOutDataTypeStr=Inherit: Inherit via back propagation  ClampingZeroOutMin=[]  ClampingZeroOutMax=[]  FilterDenConstantOutDataTypeStr=Inherit: Inherit via back propagation  FilterDenConstantOutMin=[]  FilterDenConstantOutMax=[]  PCopyOutDataTypeStr=Inherit: Inherit via back propagation  PCopyOutMin=[]  PCopyOutMax=[]  NCopyOutDataTypeStr=Inherit: Inherit via back propagation  NCopyOutMin=[]  NCopyOutMax=[]  IntegratorContinuousStateAttributes=''  IntegratorStateMustResolveToSignalObject=off  IntegratorRTWStateStorageClass=Auto  FilterContinuousStateAttributes=''  FilterStateMustResolveToSignalObject=off  FilterRTWStateStorageClass=Auto  ParallelPVariant=InternalParameters  IdealPVariant=Disabled  IVariant=InternalParameters  DVariant=InternalParameters  IntegratorVariant=Continuous  SatVariant=Disabled  AWVariant=Passthrough  PCopyVariant=Disabled  TRVariant=Disabled  FdbkBlocksVariant=Forward  IdealPFdbkVariant=Disabled  SatFdbkVariant=Disabled  DerivativeFilterVariant=ContFilter  NVariant=InternalParameters  NCopyVariant=Disabled  FilterICVariant=InternalICsFilter  IntegratorICVariant=InternalICs  ExternalResetVariant=Disabled  TRSumVariant=Passthrough  SumFdbkVariant=Disabled  SumVariant=Sum_PID  TsampFilterVariant=InternalTs  TsampNgainVariant=Passthrough  TsampIntegralVariant=Disabled_SignalSpec  ExternalSaturationOutDataTypeStr=Inherit: Same as second input  DerivativeSourceVariant=ErrorSignal
  Lateral_Vel_Control : slpidlib/PID Controller  Controller=PI  Form=Parallel  TimeDomain=Continuous-time  UseExternalTs=off  SampleTime=-1  IntegratorMethod=Forward Euler  FilterMethod=Forward Euler  ControllerParametersSource=internal  P=Kp_LatVel  I=Ki_LatVel  UseKiTs=off  D=0  UseExternalDerivativeSource=off  N=100  UseFilter=on  TunerSelectOption=Transfer Function Based (PID Tuner App)  InitialConditionSource=internal  InitialConditionForIntegrator=0  InitialConditionForFilter=0  DifferentiatorICPrevScaledInput=0  ExternalReset=none  TrackingMode=off  Kt=1  LimitOutput=off  SatLimitsSource=internal  UpperSaturationLimit=inf  LowerSaturationLimit=-inf  LinearizeAsGain=on  AntiWindupMode=none  Kb=1  LimitIntegrator=off  UpperIntegratorSaturationLimit=inf  LowerIntegratorSaturationLimit=-inf  POutMin=[]  POutMax=[]  IOutMin=[]  IOutMax=[]  DOutMin=[]  DOutMax=[]  NOutMin=[]  NOutMax=[]  SumOutMin=[]  SumOutMax=[]  SaturationOutMin=[]  SaturationOutMax=[]  PParamMin=[]  PParamMax=[]  IParamMin=[]  IParamMax=[]  DParamMin=[]  DParamMax=[]  NParamMin=[]  NParamMax=[]  KbParamMin=[]  KbParamMax=[]  KtParamMin=[]  KtParamMax=[]  KbOutMin=[]  KbOutMax=[]  KtOutMin=[]  KtOutMax=[]  IntegratorOutMin=[]  IntegratorOutMax=[]  FilterOutMin=[]  FilterOutMax=[]  SumI1OutMin=[]  SumI1OutMax=[]  SumI2OutMin=[]  SumI2OutMax=[]  SumI3OutMin=[]  SumI3OutMax=[]  SumI4OutMin=[]  SumI4OutMax=[]  SumDOutMin=[]  SumDOutMax=[]  DifferentiatorOutMin=[]  DifferentiatorOutMax=[]  FilterDiffOutCoefMin=[]  FilterDiffOutCoefMax=[]  ReciprocalOutMin=[]  ReciprocalOutMax=[]  SumDenOutMin=[]  SumDenOutMax=[]  SumNumOutMin=[]  SumNumOutMax=[]  DivideOutMin=[]  DivideOutMax=[]  UdiffTsProdOutMin=[]  UdiffTsProdOutMax=[]  NTsProdOutMin=[]  NTsProdOutMax=[]  UintegralTsProdOutMin=[]  UintegralTsProdOutMax=[]  UngainTsProdOutMin=[]  UngainTsProdOutMax=[]  ClampingZeroOutDataTypeStr=Inherit: Inherit via back propagation  ClampingZeroOutMin=[]  ClampingZeroOutMax=[]  FilterDenConstantOutDataTypeStr=Inherit: Inherit via back propagation  FilterDenConstantOutMin=[]  FilterDenConstantOutMax=[]  PCopyOutDataTypeStr=Inherit: Inherit via back propagation  PCopyOutMin=[]  PCopyOutMax=[]  NCopyOutDataTypeStr=Inherit: Inherit via back propagation  NCopyOutMin=[]  NCopyOutMax=[]  IntegratorContinuousStateAttributes=''  IntegratorStateMustResolveToSignalObject=off  IntegratorRTWStateStorageClass=Auto  FilterContinuousStateAttributes=''  FilterStateMustResolveToSignalObject=off  FilterRTWStateStorageClass=Auto  ParallelPVariant=InternalParameters  IdealPVariant=Disabled  IVariant=InternalParameters  DVariant=Disabled  IntegratorVariant=Continuous  SatVariant=Disabled  AWVariant=Passthrough  PCopyVariant=Disabled  TRVariant=Disabled  FdbkBlocksVariant=Forward  IdealPFdbkVariant=Disabled  SatFdbkVariant=Disabled  DerivativeFilterVariant=Disabled  NVariant=Disabled  NCopyVariant=Disabled_SignalSpec  FilterICVariant=Disabled  IntegratorICVariant=InternalICs  ExternalResetVariant=Disabled  TRSumVariant=Passthrough  SumFdbkVariant=Disabled  SumVariant=Sum_PI  TsampFilterVariant=InternalTs  TsampNgainVariant=Passthrough  TsampIntegralVariant=Disabled_SignalSpec  ExternalSaturationOutDataTypeStr=Inherit: Same as second input  DerivativeSourceVariant=Disabled
  Negate34 : Gain  Gain=-1
  PID Controller (2DOF) : slpidlib/PID Controller (2DOF)  Controller=PID  Form=Parallel  TimeDomain=Continuous-time  UseExternalTs=off  SampleTime=-1  IntegratorMethod=Forward Euler  FilterMethod=Forward Euler  ControllerParametersSource=internal  P=1.5256065337802  I=0.0199462340716751  UseKiTs=off  D=0.641893163639143  UseExternalDerivativeSource=off  N=15.7606402309303  UseFilter=on  b=0.994537870837311  c=0.0133325990066141  TunerSelectOption=Frequency Response Based  InitialConditionSource=internal  InitialConditionForIntegrator=0  InitialConditionForFilter=0  DifferentiatorICPrevScaledInput=0  ExternalReset=none  TrackingMode=off  Kt=1  LimitOutput=on  SatLimitsSource=internal  UpperSaturationLimit=inf  LowerSaturationLimit=-inf  LinearizeAsGain=on  AntiWindupMode=clamping  Kb=1  LimitIntegrator=on  UpperIntegratorSaturationLimit=vCmd_Integr_Limit  LowerIntegratorSaturationLimit=-vCmd_Integr_Limit  POutMin=[]  POutMax=[]  IOutMin=[]  IOutMax=[]  DOutMin=[]  DOutMax=[]  NOutMin=[]  NOutMax=[]  bOutMin=[]  bOutMax=[]  cOutMin=[]  cOutMax=[]  SumOutMin=[]  SumOutMax=[]  SaturationOutMin=[]  SaturationOutMax=[]  PParamMin=[]  PParamMax=[]  IParamMin=[]  IParamMax=[]  DParamMin=[]  DParamMax=[]  NParamMin=[]  NParamMax=[]  bParamMin=[]  bParamMax=[]  cParamMin=[]  cParamMax=[]  KbParamMin=[]  KbParamMax=[]  KtParamMin=[]  KtParamMax=[]  KbOutMin=[]  KbOutMax=[]  KtOutMin=[]  KtOutMax=[]  IntegratorOutMin=[]  IntegratorOutMax=[]  FilterOutMin=[]  FilterOutMax=[]  SumI1OutMin=[]  SumI1OutMax=[]  SumI2OutMin=[]  SumI2OutMax=[]  SumI3OutMin=[]  SumI3OutMax=[]  SumI4OutMin=[]  SumI4OutMax=[]  SumDOutMin=[]  SumDOutMax=[]  Sum1OutMin=[]  Sum1OutMax=[]  Sum2OutMin=[]  Sum2OutMax=[]  Sum3OutMin=[]  Sum3OutMax=[]  DifferentiatorOutMin=[]  DifferentiatorOutMax=[]  FilterDiffOutCoefMin=[]  FilterDiffOutCoefMax=[]  ReciprocalOutMin=[]  ReciprocalOutMax=[]  SumDenOutMin=[]  SumDenOutMax=[]  SumNumOutMin=[]  SumNumOutMax=[]  DivideOutMin=[]  DivideOutMax=[]  UdiffTsProdOutMin=[]  UdiffTsProdOutMax=[]  NTsProdOutMin=[]  NTsProdOutMax=[]  UintegralTsProdOutMin=[]  UintegralTsProdOutMax=[]  UngainTsProdOutMin=[]  UngainTsProdOutMax=[]  ClampingZeroOutDataTypeStr=Inherit: Inherit via back propagation  ClampingZeroOutMin=[]  ClampingZeroOutMax=[]  FilterDenConstantOutDataTypeStr=Inherit: Inherit via back propagation  FilterDenConstantOutMin=[]  FilterDenConstantOutMax=[]  PCopyOutDataTypeStr=Inherit: Inherit via back propagation  PCopyOutMin=[]  PCopyOutMax=[]  NCopyOutDataTypeStr=Inherit: Inherit via back propagation  NCopyOutMin=[]  NCopyOutMax=[]  IntegratorContinuousStateAttributes=''  IntegratorStateMustResolveToSignalObject=off  IntegratorRTWStateStorageClass=Auto  FilterContinuousStateAttributes=''  FilterStateMustResolveToSignalObject=off  FilterRTWStateStorageClass=Auto  ParallelPVariant=InternalParameters  IdealPVariant=Disabled  IVariant=InternalParameters  DVariant=InternalParameters  bVariant=InternalParameters  cVariant=InternalParameters  IntegratorVariant=Continuous  SatVariant=Enabled  AWVariant=ContClampingParallel  PCopyVariant=Disabled  TRVariant=Disabled  FdbkBlocksVariant=Forward  IdealPFdbkVariant=Disabled  SatFdbkVariant=Disabled  DerivativeFilterVariant=ContFilter  NVariant=InternalParameters  NCopyVariant=Disabled  FilterICVariant=InternalICsFilter  IntegratorICVariant=InternalICs  ExternalResetVariant=Disabled  TRSumVariant=Passthrough  SumFdbkVariant=Disabled  SumVariant=Sum_PID  TsampFilterVariant=InternalTs  TsampNgainVariant=Passthrough  TsampIntegralVariant=Disabled_SignalSpec  ExternalSaturationOutDataTypeStr=Inherit: Same as second input  DerivativeSourceVariant=ErrorSignal
  Pitch_Limit : Saturate  UpperLimit=pitch_Cmd_Limit  LowerLimit=-pitch_Cmd_Limit
  Pitch_PD_ Controller : slpidlib/PID Controller  Controller=PD  Form=Parallel  TimeDomain=Continuous-time  UseExternalTs=off  SampleTime=-1  IntegratorMethod=Forward Euler  FilterMethod=Forward Euler  ControllerParametersSource=internal  P=Kp_Pitch  I=1  UseKiTs=off  D=Kd_Pitch  UseExternalDerivativeSource=off  N=N_Pitch  UseFilter=on  TunerSelectOption=Transfer Function Based (PID Tuner App)  InitialConditionSource=internal  InitialConditionForIntegrator=0  InitialConditionForFilter=0  DifferentiatorICPrevScaledInput=0  ExternalReset=none  TrackingMode=off  Kt=1  LimitOutput=off  SatLimitsSource=internal  UpperSaturationLimit=inf  LowerSaturationLimit=-inf  LinearizeAsGain=on  AntiWindupMode=none  Kb=1  LimitIntegrator=off  UpperIntegratorSaturationLimit=inf  LowerIntegratorSaturationLimit=-inf  POutMin=[]  POutMax=[]  IOutMin=[]  IOutMax=[]  DOutMin=[]  DOutMax=[]  NOutMin=[]  NOutMax=[]  SumOutMin=[]  SumOutMax=[]  SaturationOutMin=[]  SaturationOutMax=[]  PParamMin=[]  PParamMax=[]  IParamMin=[]  IParamMax=[]  DParamMin=[]  DParamMax=[]  NParamMin=[]  NParamMax=[]  KbParamMin=[]  KbParamMax=[]  KtParamMin=[]  KtParamMax=[]  KbOutMin=[]  KbOutMax=[]  KtOutMin=[]  KtOutMax=[]  IntegratorOutMin=[]  IntegratorOutMax=[]  FilterOutMin=[]  FilterOutMax=[]  SumI1OutMin=[]  SumI1OutMax=[]  SumI2OutMin=[]  SumI2OutMax=[]  SumI3OutMin=[]  SumI3OutMax=[]  SumI4OutMin=[]  SumI4OutMax=[]  SumDOutMin=[]  SumDOutMax=[]  DifferentiatorOutMin=[]  DifferentiatorOutMax=[]  FilterDiffOutCoefMin=[]  FilterDiffOutCoefMax=[]  ReciprocalOutMin=[]  ReciprocalOutMax=[]  SumDenOutMin=[]  SumDenOutMax=[]  SumNumOutMin=[]  SumNumOutMax=[]  DivideOutMin=[]  DivideOutMax=[]  UdiffTsProdOutMin=[]  UdiffTsProdOutMax=[]  NTsProdOutMin=[]  NTsProdOutMax=[]  UintegralTsProdOutMin=[]  UintegralTsProdOutMax=[]  UngainTsProdOutMin=[]  UngainTsProdOutMax=[]  ClampingZeroOutDataTypeStr=Inherit: Inherit via back propagation  ClampingZeroOutMin=[]  ClampingZeroOutMax=[]  FilterDenConstantOutDataTypeStr=Inherit: Inherit via back propagation  FilterDenConstantOutMin=[]  FilterDenConstantOutMax=[]  PCopyOutDataTypeStr=Inherit: Inherit via back propagation  PCopyOutMin=[]  PCopyOutMax=[]  NCopyOutDataTypeStr=Inherit: Inherit via back propagation  NCopyOutMin=[]  NCopyOutMax=[]  IntegratorContinuousStateAttributes=''  IntegratorStateMustResolveToSignalObject=off  IntegratorRTWStateStorageClass=Auto  FilterContinuousStateAttributes=''  FilterStateMustResolveToSignalObject=off  FilterRTWStateStorageClass=Auto  ParallelPVariant=InternalParameters  IdealPVariant=Disabled  IVariant=Disabled  DVariant=InternalParameters  IntegratorVariant=Disabled  SatVariant=Disabled  AWVariant=Disabled  PCopyVariant=Disabled  TRVariant=Disabled  FdbkBlocksVariant=Forward  IdealPFdbkVariant=Disabled  SatFdbkVariant=Disabled  DerivativeFilterVariant=ContFilter  NVariant=InternalParameters  NCopyVariant=Disabled  FilterICVariant=InternalICsFilter  IntegratorICVariant=Disabled  ExternalResetVariant=Disabled  TRSumVariant=Passthrough  SumFdbkVariant=Disabled  SumVariant=Sum_PD  TsampFilterVariant=InternalTs  TsampNgainVariant=Passthrough  TsampIntegralVariant=Disabled_SignalSpec  ExternalSaturationOutDataTypeStr=Inherit: Same as second input  DerivativeSourceVariant=ErrorSignal
  Spread_Out : Gain  Gain=1/nFans
  Sum{,1..3} (4 alike) : Sum
  Sum4 : Sum  Inputs=|+-
  Sum5 : Sum  Inputs=|++
  Sum8 : Sum  Inputs=|+-
  Terminator : Terminator
  To Workspace : ToWorkspace  VariableName=vLimit  SaveFormat=Timeseries  SampleTime=-1
  VcmdX : Scope  Commented=on  NumInputPorts=2
  VcmdX1 : Scope  Commented=on  NumInputPorts=2
  Velocity_Limit : Saturate  UpperLimit=velCmd_Limit  LowerLimit=-velCmd_Limit
  Y_intercept : Constant  Value=bOmega
  slope : Gain  Gain=mOmega
  xCmd : Outport
  yCmd : Outport  Port=2
  Omega_Cmds : Outport  Port=3
  wires:
  Clock/1 -> Lateral_Flight_Plan/1(t)
  Lateral_Flight_Plan/2(xCmd) -> Filter_Cmd1/1(xC), xCmd/1, VcmdX1/1
  Gain2/1 -> Gain1/1
  Sum3/1 -> Bus Creator2/4  "M4"
  Negate34/1 -> Sum3/1, Sum2/2
  Gain1/1 -> slope/1
  Bus Creator2/1 -> Omega_Cmds/1
  slope/1 -> Sum5/1
  Sum1/1 -> Bus Creator2/1  "M1"
  Sum5/1 -> Sum3/2, Sum2/1, Sum1/1, Sum/2
  Y_intercept/1 -> Sum5/2
  Sum/1 -> Bus Creator2/2  "M2"
  m/1 -> Gain/1
  Cosine_Loss/1 -> Gain2/1
  Gain/1 -> Cosine_Loss/1
  Spread_Out/1 -> [Pitch_Omega]
  [Pitch_Omega] -> Sum/1, Sum1/2
  Sum2/1 -> Bus Creator2/3  "M3"
  [Pitch_Omega] -> Negate34/1
  Sched_Lateral/1 -> Lateral_Flight_Plan/2(LatFlt_Schedule)
  Lateral_Flight_Plan/1(modeLat) -> Terminator/1
  Lateral_Flight_Plan/3(vLim) -> To Workspace/1
  Vx/1 -> Sum4/2
  Sum4/1 -> Lateral_Vel_Control/1
  Lateral_Vel_Control/1 -> Sum8/1
  Sum8/1 -> Pitch_Limit/1
  Theta/1 -> Sum8/2
  Velocity_Limit/1 -> VcmdX/2, Sum4/1
  Pitch_PD_ Controller/1 -> Spread_Out/1
  PID Controller (2DOF)/1 -> VcmdX/1, Velocity_Limit/1
  Filter_Cmd1/1(xC_F) -> PID Controller (2DOF)/1, VcmdX1/2
  x/1 -> PID Controller (2DOF)/2
  Pitch_Limit/1 -> Pitch_PD_ Controller/1
  Constant/1 -> yCmd/1
